simulink model "SWC_FDC_type"  (R2021b)
settings: Solver=FixedStepDiscrete  StartTime=0.0  StopTime=10.0  FixedStep=0.001  RelTol=1e-3
values from neighbouring files (symbols this model uses):
  DID_VCUKey = uint16(0x0202)    [vcu_local_hdr.m]
  DID_XWD = uint16(513)    [vcu_local_hdr.m]
  DIDLen_APSFunConfig = uint16(16)    [vcu_local_hdr.m]
  DIDLen_AutoLock = uint16(1)    [vcu_local_hdr.m]
  DIDLen_DKCKey = uint16(8)    [vcu_local_hdr.m]
  DIDLen_DRLDis = uint16(1)    [vcu_local_hdr.m]
  DIDLen_DynoMode = uint16(1)    [vcu_local_hdr.m]
  DIDLen_FMHTimer = uint16(1)    [vcu_local_hdr.m]
  DIDLen_LFLowPresThre = uint16(1)    [vcu_local_hdr.m]
  DIDLen_LFSensorID = uint16(4)    [vcu_local_hdr.m]
  DIDLen_LRLowPresThre = uint16(1)    [vcu_local_hdr.m]
  DIDLen_LRSensorID = uint16(4)    [vcu_local_hdr.m]
  DIDLen_RFLowPresThre = uint16(1)    [vcu_local_hdr.m]
  DIDLen_RFSensorID = uint16(4)    [vcu_local_hdr.m]
  DIDLen_RRLowPresThre = uint16(1)    [vcu_local_hdr.m]
  DIDLen_RRSensorID = uint16(4)    [vcu_local_hdr.m]
  DIDLen_SensorMode = uint16(1)    [vcu_local_hdr.m]
  DIDLen_TireSize = uint16(16)    [vcu_local_hdr.m]
  DIDLen_TPMSLearnSta = uint16(1)    [vcu_local_hdr.m]
  DIDLen_TurnLampFLThreCurr = uint16(1)    [vcu_local_hdr.m]
  DIDLen_TurnLampFRThreCurr = uint16(1)    [vcu_local_hdr.m]
  DIDLen_TurnLampRLThreCurr = uint16(1)    [vcu_local_hdr.m]
  DIDLen_TurnLampRRThreCurr = uint16(1)    [vcu_local_hdr.m]
  DIDLen_USSConfig = uint16(16)    [vcu_local_hdr.m]
  DIDLen_WhlPres = uint16(4)    [vcu_local_hdr.m]
  DIDLen_WhlSensorBattSta = uint16(1)    [vcu_local_hdr.m]
  DIDLen_WhlTmp = uint16(4)    [vcu_local_hdr.m]
  DIDLen_XWDMode = uint16(1)    [vcu_local_hdr.m]
  DIDNum_APSFunConfig = uint16(0x0903)    [vcu_local_hdr.m]
  DIDNum_AutoLock = uint16(0x0306)    [vcu_local_hdr.m]
  DIDNum_DKCKey = uint16(0x0202)    [vcu_local_hdr.m]
  DIDNum_DRLDis = uint16(0x0307)    [vcu_local_hdr.m]
  DIDNum_DynoMode = uint16(0x0203)    [vcu_local_hdr.m]
  DIDNum_FMHTimer = uint16(0x0305)    [vcu_local_hdr.m]
  DIDNum_LFLowPresThre = uint16(0x0B08)    [vcu_local_hdr.m]
  DIDNum_LFSensorID = uint16(0x0B01)    [vcu_local_hdr.m]
  DIDNum_LRLowPresThre = uint16(0x0B0A)    [vcu_local_hdr.m]
  DIDNum_LRSensorID = uint16(0x0B03)    [vcu_local_hdr.m]
  DIDNum_RFLowPresThre = uint16(0x0B09)    [vcu_local_hdr.m]
  DIDNum_RFSensorID = uint16(0x0B02)    [vcu_local_hdr.m]
  DIDNum_RRLowPresThre = uint16(0x0B0B)    [vcu_local_hdr.m]
  DIDNum_RRSensorID = uint16(0x0B04)    [vcu_local_hdr.m]
  DIDNum_SensorMode = uint16(0x0B0C)    [vcu_local_hdr.m]
  DIDNum_TireSize = uint16(0x0902)    [vcu_local_hdr.m]
  DIDNum_TPMSLearnSta = uint16(0x0B0D)    [vcu_local_hdr.m]
  DIDNum_TurnLampFLThreCurr = uint16(0x0303)    [vcu_local_hdr.m]
  DIDNum_TurnLampFRThreCurr = uint16(0x0301)    [vcu_local_hdr.m]
  DIDNum_TurnLampRLThreCurr = uint16(0x0304)    [vcu_local_hdr.m]
  DIDNum_TurnLampRRThreCurr = uint16(0x0302)    [vcu_local_hdr.m]
  DIDNum_USSConfig = uint16(0x0901)    [vcu_local_hdr.m]
  DIDNum_WhlPres = uint16(0x0B05)    [vcu_local_hdr.m]
  DIDNum_WhlSensorBattSta = uint16(0x0B07)    [vcu_local_hdr.m]
  DIDNum_WhlTmp = uint16(0x0B06)    [vcu_local_hdr.m]
  DIDNum_XWDMode = uint16(0x0201)    [vcu_local_hdr.m]
  DIDVCUKeyLength = uint16(8)    [vcu_local_hdr.m]
  ENUM_DRIVETRAIN_AWD = uint8(  2  )    [vcu_local_hdr.m]
  ENUM_DRIVETRAIN_FWD = uint8(  1  )    [vcu_local_hdr.m]
  ENUM_DRIVETRAIN_RWD = uint8(  0  )    [vcu_local_hdr.m]
  ENUM_TPMSLearnStatus_LEARNED = uint8(  1  )    [vcu_local_hdr.m]
  ENUM_TPMSLearnStatus_LEARNFAIL = uint8(  2  )    [vcu_local_hdr.m]
  ENUM_TPMSLearnStatus_NOTLEARN = uint8(  0  )    [vcu_local_hdr.m]
  ENUM_TPMSSTA_FAT = uint8(  8  )    [vcu_local_hdr.m]
  ENUM_TPMSSTA_LOWBATTERY = uint8(  2  )    [vcu_local_hdr.m]
  FALSE = boolean( 0 )    [vcu_local_hdr.m]
  ONE_INT = uint8(1)    [vcu_local_hdr.m]
  P_boolean = 0.0    [APPTypes.sldd]
  TRUE = boolean( 1 )    [vcu_local_hdr.m]
  ZERO_FLOAT = single(0)    [vcu_local_hdr.m]
  ZERO_INT = uint8(0)    [vcu_local_hdr.m]
undefined symbols (not defined in the file or in its folder): f32_ApsOutVehSpdSig, KHAL_DKCDecryptEnable_flg_ovrdflg, KHAL_DKCDecryptEnable_flg_ovrdval, KHAL_RandomNumberY1_enum, KHAL_RandomNumberY2_enum, KHAL_RandomNumberY_ovrdflg, KHAL_TPMSRESBUTT_flg_ovrdflg, KHAL_TPMSRESBUTT_flg_ovrdval, R_DIDWriteCDD_CSOP_DIDSet_APSFunConfig, R_DIDWriteCDD_CSOP_DIDSet_AutoLock, R_DIDWriteCDD_CSOP_DIDSet_DKCKey, R_DIDWriteCDD_CSOP_DIDSet_DRLDis, R_DIDWriteCDD_CSOP_DIDSet_DynoMode, R_DIDWriteCDD_CSOP_DIDSet_FMHTimer, R_DIDWriteCDD_CSOP_DIDSet_LFLowPresThre, R_DIDWriteCDD_CSOP_DIDSet_LFSensorID, R_DIDWriteCDD_CSOP_DIDSet_LRLowPresThre, R_DIDWriteCDD_CSOP_DIDSet_LRSensorID, R_DIDWriteCDD_CSOP_DIDSet_RFLowPresThre, R_DIDWriteCDD_CSOP_DIDSet_RFSensorID, R_DIDWriteCDD_CSOP_DIDSet_RRLowPresThre, R_DIDWriteCDD_CSOP_DIDSet_RRSensorID, R_DIDWriteCDD_CSOP_DIDSet_SensorMode, R_DIDWriteCDD_CSOP_DIDSet_TireSize, R_DIDWriteCDD_CSOP_DIDSet_TPMSLearnSta, R_DIDWriteCDD_CSOP_DIDSet_TurnLampFLThreCurr, R_DIDWriteCDD_CSOP_DIDSet_TurnLampFRThreCurr, R_DIDWriteCDD_CSOP_DIDSet_TurnLampRLThreCurr, R_DIDWriteCDD_CSOP_DIDSet_TurnLampRRThreCurr, R_DIDWriteCDD_CSOP_DIDSet_USSConfig, R_DIDWriteCDD_CSOP_DIDSet_WhlPres, R_DIDWriteCDD_CSOP_DIDSet_WhlSensorBattSta, R_DIDWriteCDD_CSOP_DIDSet_WhlTmp, R_DIDWriteCDD_CSOP_DIDSet_XWDMode, R_E2E_CAN3_VCU1_CSOP_Write_CAN3_VCU1, R_E2E_CAN3_VCU1_toNIDEC_CSOP_Write_CAN3_VCU1_toNIDEC, R_E2E_CAN4_VCU1_CSOP_Write_CAN4_VCU1, R_FDCCDD_Inner_CSOP_FDC_AppCallSleep, R_HALINCDD_CSOP_PAS_Handler, R_HALINCDD_CSOP_UDS_Main, R_HALOUT_APS_CSOP_ApsOutput, R_HALOUTCDD_CSOP_AppNmStateReq, R_HALOUTCDD_CSOP_SetAcoreRebootCmdACK, R_HALOUTCDD_CSOP_SetSysPwrStat, R_HALOUTCDD_CSOP_SleepRequest, R_IOExpOUT_CDD_CSOP_IOExpSetVal, R_J1939_CAN1_CFGEM1_BAM_CSOP_Write_CAN1_CFGEM1_BAM, R_J1939_CAN1_CFGEM1_DT_CSOP_Write_CAN1_CFGEM1_DT, R_NVMReadCDD_Inner_NVM_ReadOperation, R_NVMWriteCDD_Inner_NVM_WriteOperation, R_UDSCDD_CSOP_DdmRestartOperationCycle, R_WDGCDD_CSOP_Call_Watchdog, R_WDGCDD_CSOP_Call_WDG_AppEnd, R_WDGCDD_CSOP_Call_WDG_AppStart, u16_DIDLen_APSFunConfig, u16_DIDLen_AutoLock, u16_DIDLen_DKCKey, u16_DIDLen_DRLDis, u16_DIDLen_DynoMode, u16_DIDLen_FMHTimer ... (+83)
libraries: simulink x215, FVT_lib x143, hcu_lib x19, hdlsllib x9, app x1, halin x1, halout x1, inp x1, outp x1
(part 1 of 13)
settings Model: DataDictionary=APPTypes.sldd  Creator=FVT22063  LastModifiedBy=FVT22063
settings DataIOCC: SaveFormat=StructureWithTime
settings OptimizationCC: DefaultParameterBehavior=Inlined  EnhancedBackFolding=on  PassReuseOutputArgsAs=Individual arguments  ZeroExternalMemoryAtStartup=off  ZeroInternalMemoryAtStartup=off  OptimizeBlockOrder=speed  DifferentSizesBufferReuse=on  OptimizationCustomize=off  EfficientTunableParamExpr=on
settings DebuggingCC: ParameterTunabilityLossMsg=error
settings HardwareCC: ProdBitPerPointer=32  ProdBitPerSizeT=32  ProdBitPerPtrDiffT=32  ProdLargestAtomicInteger=Long  ProdLargestAtomicFloat=Double  ProdWordSize=32  ProdLongLongMode=on  ProdHWDeviceType=ARM Compatible->ARM Cortex-M
settings ModelReferenceCC: ModelReferenceNumInstancesAllowed=Single
settings SFSimCC: MATLABDynamicMemAlloc=off
settings RTWCC: Description=AUTOSAR  SystemTargetFile=autosar.tlc  GenCodeOnly=on  TemplateMakefile=ert_default_tmf  PortableWordSizes=on
settings CodeAppCC: ForceParamTrailComments=on  IgnoreCustomStorageClasses=off  OperatorAnnotations=on  SimulinkDataObjDesc=on  SFDataObjDesc=on  InsertBlockDesc=on
settings STFCustomTargetCC: TargetLangStandard=C99 (ISO)  MultiwordLength=256  ParMdlRefBuildCompliant=on  CompOptLevelCompliant=on  IncludeMdlTerminateFcn=off  CombineOutputUpdateFcns=on  SuppressErrorStatus=on  ERTCustomFileBanners=on  SupportNonFinite=off  SupportComplex=off  SupportContinuousTime=off  SupportNonInlinedSFcns=off  RemoveResetFunc=on  MATLABClassNameForMDSCustomization=Simulink.SoftwareTarget.ERTCustomization  AutosarCompliant=on  GRTInterface=off  UseToolchainInfoCompliant=on  LookupTableObjectStructAxisOrder=2,1,3,4,...  LUTObjectStructOrderEvenSpacing=Size,Table,Breakpoints  SystemTargetFile=autosar.tlc
settings ERTTargetCC: TargetLangStandard=C99 (ISO)  ConcurrentExecutionCompliant=off  IncludeMdlTerminateFcn=off  SuppressErrorStatus=on  SupportNonFinite=off  SupportComplex=off  ModelStepFunctionPrototypeControlCompliant=off  CPPClassGenCompliant=off  AutosarCompliant=on  LookupTableObjectStructAxisOrder=2,1,3,4,...  LUTObjectStructOrderEvenSpacing=Size,Table,Breakpoints  GenerateASAP2=on  InlinedParameterPlacement=NonHierarchical  ERTCustomFileTemplate=example_file_process.tlc  ConvertIfToSwitch=off  SuppressUnreachableDefaultCases=off  BooleanTrueId=true_MatlabRTW  BooleanFalseId=false_MatlabRTW

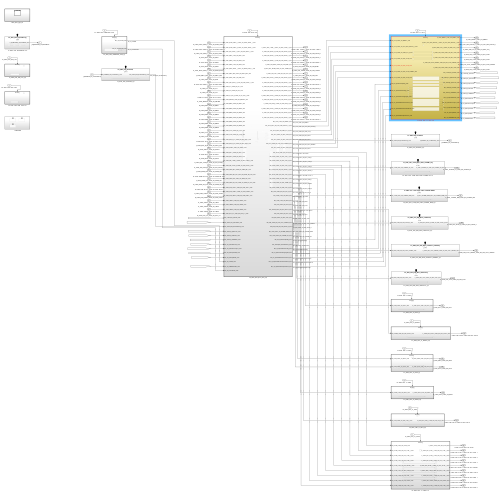
[thumbnail: Simulink's stored preview of the top-level diagram]
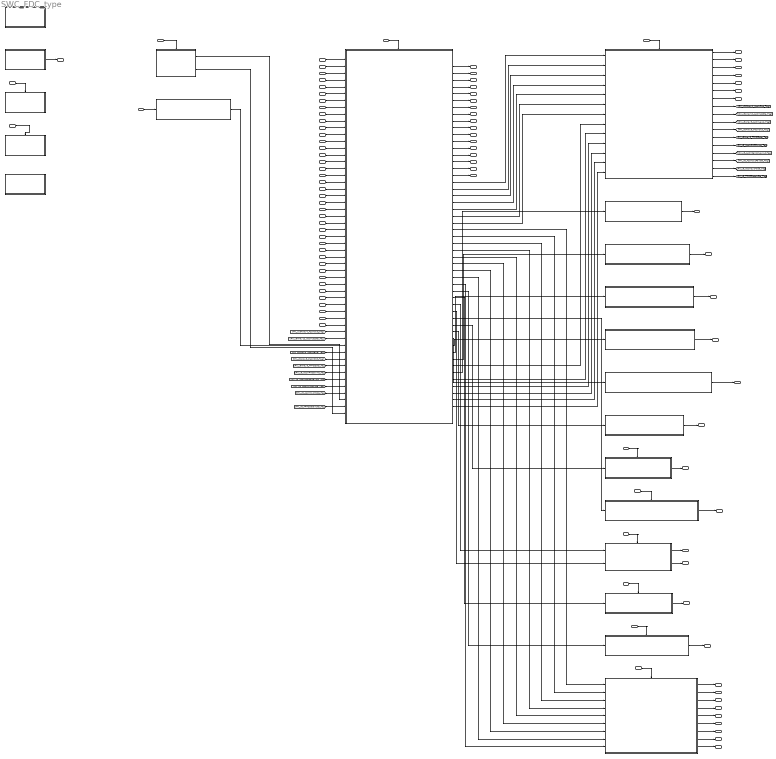
== system SWC_FDC_type ==
  run_SWC_FDC_PAS_1ms : Inport  SampleTime=0.001  OutputFunctionCall=on
  run_SWC_FDC_UDS_10ms : Inport  Port=2  SampleTime=0.01  OutputFunctionCall=on
  run_SWC_FDC_IOEXPCDD_10ms : Inport  Port=3  SampleTime=0.01  OutputFunctionCall=on
  run_SWC_FDC_RxTx_5ms : Inport  Port=4  SampleTime=0.005  OutputFunctionCall=on
  run_SWC_FDC_Tx_10ms : Inport  Port=5  SampleTime=0.01  OutputFunctionCall=on
  run_SWC_FDC_Tx_80ms : Inport  Port=6  SampleTime=0.08  OutputFunctionCall=on
  run_SWC_FDC_Tx_5000ms : Inport  Port=7  SampleTime=5  OutputFunctionCall=on
  run_SWC_FDC_Tx_50ms : Inport  Port=8  SampleTime=0.05  OutputFunctionCall=on
  run_SWC_FDC_Tx_250ms : Inport  Port=9  SampleTime=0.25  OutputFunctionCall=on
  run_SWC_FDC_Tx_20ms : Inport  Port=10  SampleTime=0.02  OutputFunctionCall=on
  run_SWC_FDC_Tx_100ms : Inport  Port=11  SampleTime=0.1  OutputFunctionCall=on
  R_NVMRead_NV_FVTDataArray : Inport  Port=12  OutDataTypeStr=uint8  PortDimensions=256
  R_CAN1_DCDC_Status_1_CAN1_SG_DCDC_Status_1 : Inport  Port=13  OutDataTypeStr=Bus: DT_CAN1_SG_DCDC_Status_1  PortDimensions=1  BusOutputAsStruct=on
  R_CAN1_DCDC_Status_2_CAN1_SG_DCDC_Status_2 : Inport  Port=14  OutDataTypeStr=Bus: DT_CAN1_SG_DCDC_Status_2  PortDimensions=1  BusOutputAsStruct=on
  R_CAN1_EAC_Status_1_CAN1_SG_EAC_Status_1 : Inport  Port=15  OutDataTypeStr=Bus: DT_CAN1_SG_EAC_Status_1  PortDimensions=1  BusOutputAsStruct=on
  R_CAN1_EBC1_CAN1_SG_EBC1 : Inport  Port=16  OutDataTypeStr=Bus: DT_CAN1_SG_EBC1  PortDimensions=1  BusOutputAsStruct=on
  R_CAN1_EBC2_CAN1_SG_EBC2 : Inport  Port=17  OutDataTypeStr=Bus: DT_CAN1_SG_EBC2  PortDimensions=1  BusOutputAsStruct=on
  R_CAN1_EBC5_CAN1_SG_EBC5 : Inport  Port=18  OutDataTypeStr=Bus: DT_CAN1_SG_EBC5  PortDimensions=1  BusOutputAsStruct=on
  R_CAN1_EHPS_Status_1_CAN1_SG_EHPS_Status_1 : Inport  Port=19  OutDataTypeStr=Bus: DT_CAN1_SG_EHPS_Status_1  PortDimensions=1  BusOutputAsStruct=on
  R_CAN1_EMC1_EM1_CAN1_SG_EMC1_EM1 : Inport  Port=20  OutDataTypeStr=Bus: DT_CAN1_SG_EMC1_EM1  PortDimensions=1  BusOutputAsStruct=on
  R_CAN1_EPB1_CAN1_SG_EPB1 : Inport  Port=21  OutDataTypeStr=Bus: DT_CAN1_SG_EPB1  PortDimensions=1  BusOutputAsStruct=on
  R_CAN1_PDU_Status_1_CAN1_SG_PDU_Status_1 : Inport  Port=22  OutDataTypeStr=Bus: DT_CAN1_SG_PDU_Status_1  PortDimensions=1  BusOutputAsStruct=on
  R_CAN2_IVI1_CAN2_SG_IVI1 : Inport  Port=23  OutDataTypeStr=Bus: DT_CAN2_SG_IVI1  PortDimensions=1  BusOutputAsStruct=on
  R_CAN2_IVI2_CAN2_SG_IVI2 : Inport  Port=24  OutDataTypeStr=Bus: DT_CAN2_SG_IVI2  PortDimensions=1  BusOutputAsStruct=on
  R_CAN2_IVI_P20_0_CAN2_SG_IVI_P20_0 : Inport  Port=25  OutDataTypeStr=Bus: DT_CAN2_SG_IVI_P20_0  PortDimensions=1  BusOutputAsStruct=on
  R_CAN2_METER1_CAN2_SG_METER1 : Inport  Port=26  OutDataTypeStr=Bus: DT_CAN2_SG_METER1  PortDimensions=1  BusOutputAsStruct=on
  R_CAN3_BMS1_CAN3_SG_BMS1 : Inport  Port=27  OutDataTypeStr=Bus: DT_CAN3_SG_BMS1  PortDimensions=1  BusOutputAsStruct=on
  R_CAN3_BMS3_CAN3_SG_BMS3 : Inport  Port=28  OutDataTypeStr=Bus: DT_CAN3_SG_BMS3  PortDimensions=1  BusOutputAsStruct=on
  R_CAN3_BMS4_CAN3_SG_BMS4 : Inport  Port=29  OutDataTypeStr=Bus: DT_CAN3_SG_BMS4  PortDimensions=1  BusOutputAsStruct=on
  R_CAN3_BMS5_CAN3_SG_BMS5 : Inport  Port=30  OutDataTypeStr=Bus: DT_CAN3_SG_BMS5  PortDimensions=1  BusOutputAsStruct=on
  R_CAN3_BMS6_CAN3_SG_BMS6 : Inport  Port=31  OutDataTypeStr=Bus: DT_CAN3_SG_BMS6  PortDimensions=1  BusOutputAsStruct=on
  R_CAN3_BMS8_CAN3_SG_BMS8 : Inport  Port=32  OutDataTypeStr=Bus: DT_CAN3_SG_BMS8  PortDimensions=1  BusOutputAsStruct=on
  R_CAN3_CCU1_CAN3_SG_CCU1 : Inport  Port=33  OutDataTypeStr=Bus: DT_CAN3_SG_CCU1  PortDimensions=1  BusOutputAsStruct=on
  R_CAN3_CCU2_CAN3_SG_CCU2 : Inport  Port=34  OutDataTypeStr=Bus: DT_CAN3_SG_CCU2  PortDimensions=1  BusOutputAsStruct=on
  R_CAN3_MCU_B_R1_CAN3_SG_MCU_B_R1 : Inport  Port=35  OutDataTypeStr=Bus: DT_CAN3_SG_MCU_B_R1  PortDimensions=1  BusOutputAsStruct=on
  R_CAN3_MCU_B_R2_CAN3_SG_MCU_B_R2 : Inport  Port=36  OutDataTypeStr=Bus: DT_CAN3_SG_MCU_B_R2  PortDimensions=1  BusOutputAsStruct=on
  R_CAN3_Shifter1_CAN3_SG_Shifter1 : Inport  Port=37  OutDataTypeStr=Bus: DT_CAN3_SG_Shifter1  PortDimensions=1  BusOutputAsStruct=on
  R_CAN4_DKC1_CAN4_SG_DKC1 : Inport  Port=38  OutDataTypeStr=Bus: DT_CAN4_SG_DKC1  PortDimensions=1  BusOutputAsStruct=on
  R_CAN4_DKC2_CAN4_SG_DKC2 : Inport  Port=39  OutDataTypeStr=Bus: DT_CAN4_SG_DKC2  PortDimensions=1  BusOutputAsStruct=on
  R_CAN4_Z24_C1000_0_CAN4_SG_Z24_C1000_0 : Inport  Port=40  OutDataTypeStr=Bus: DT_CAN4_SG_Z24_C1000_0  PortDimensions=1  BusOutputAsStruct=on
  R_CAN4_Z24_CE100_0_CAN4_SG_Z24_CE100_0 : Inport  Port=41  OutDataTypeStr=Bus: DT_CAN4_SG_Z24_CE100_0  PortDimensions=1  BusOutputAsStruct=on
  R_CAN4_ZONE_DR1_CAN4_SG_ZONE_DR1 : Inport  Port=42  OutDataTypeStr=Bus: DT_CAN4_SG_ZONE_DR1  PortDimensions=1  BusOutputAsStruct=on
  R_CAN4_ZONE_DR_VCU_CAN4_SG_ZONE_DR_VCU : Inport  Port=43  OutDataTypeStr=Bus: DT_CAN4_SG_ZONE_DR_VCU  PortDimensions=1  BusOutputAsStruct=on
  R_CAN4_ZONE_FR1_CAN4_SG_ZONE_FR1 : Inport  Port=44  OutDataTypeStr=Bus: DT_CAN4_SG_ZONE_FR1  PortDimensions=1  BusOutputAsStruct=on
  R_CAN4_ZONE_FR_VCU_CAN4_SG_ZONE_FR_VCU : Inport  Port=45  OutDataTypeStr=Bus: DT_CAN4_SG_ZONE_FR_VCU  PortDimensions=1  BusOutputAsStruct=on
  R_CAN4_zGW_APTC1_CAN4_SG_zGW_APTC1 : Inport  Port=46  OutDataTypeStr=Bus: DT_CAN4_SG_zGW_APTC1  PortDimensions=1  BusOutputAsStruct=on
  R_CAN4_zGW_CANFr1_CAN4_SG_zGW_CANFr1 : Inport  Port=47  OutDataTypeStr=Bus: DT_CAN4_SG_zGW_CANFr1  PortDimensions=1  BusOutputAsStruct=on
  R_CAN4_zGW_LINDr1_CAN4_SG_zGW_LINDr1 : Inport  Port=48  OutDataTypeStr=Bus: DT_CAN4_SG_zGW_LINDr1  PortDimensions=1  BusOutputAsStruct=on
  R_CAN5_TBOX1_CAN5_SG_TBOX1 : Inport  Port=49  OutDataTypeStr=Bus: DT_CAN5_SG_TBOX1  PortDimensions=1  BusOutputAsStruct=on
  R_CAN5_TBOX2_CAN5_SG_TBOX2 : Inport  Port=50  OutDataTypeStr=Bus: DT_CAN5_SG_TBOX2  PortDimensions=1  BusOutputAsStruct=on
  R_CAN5_TBOX3_CAN5_SG_TBOX3 : Inport  Port=51  OutDataTypeStr=Bus: DT_CAN5_SG_TBOX3  PortDimensions=1  BusOutputAsStruct=on
  R_CAN7_Door_Fr1_CAN7_SG_Door_Fr1 : Inport  Port=52  OutDataTypeStr=Bus: DT_CAN7_SG_Door_Fr1  PortDimensions=1  BusOutputAsStruct=on
  P_WDGCDD : Subsystem
  SWC_FDC_type_Init : Subsystem
  run_SWC_FDC_AppCallSleep_sys : Subsystem
  run_SWC_FDC_E2E_Write_CAN3VCU1_sys : Subsystem
  run_SWC_FDC_E2E_Write_CAN3VCU1_toNIDEC_sys : Subsystem
  run_SWC_FDC_E2E_Write_CAN4VCU1_sys : Subsystem
  run_SWC_FDC_IOEXPCDD_10ms_sys : Subsystem
  run_SWC_FDC_J1939_Write_CAN1_CFGEM1_BAM_sys : Subsystem
  run_SWC_FDC_J1939_Write_CAN1_CFGEM1_DT_sys : Subsystem
  run_SWC_FDC_NvmRead_sys : Subsystem
  run_SWC_FDC_NvmWrite_sys : Subsystem
  run_SWC_FDC_PAS_1ms_sys : Subsystem
  run_SWC_FDC_RxTx_5ms_sys : Subsystem
  run_SWC_FDC_Tx_100ms_sys : Subsystem
  run_SWC_FDC_Tx_10ms_sys : Subsystem
  run_SWC_FDC_Tx_20ms_sys : Subsystem
  run_SWC_FDC_Tx_250ms_sys : Subsystem
  run_SWC_FDC_Tx_5000ms_sys : Subsystem
  run_SWC_FDC_Tx_50ms_sys : Subsystem
  run_SWC_FDC_Tx_80ms_sys : Subsystem
  run_SWC_FDC_UDS_10ms_sys : Subsystem
  P_AppModeReq_requestedMode : Outport  OutDataTypeStr=Enum: AppModeRequestType  PortDimensions=1
  P_CAN1_GW1_C1000_1_CAN1_SG_GW1_C1000_1 : Outport  Port=2  OutDataTypeStr=Bus: DT_CAN1_SG_GW1_C1000_1  PortDimensions=1  BusOutputAsStruct=on
  P_CAN2_FD2_CE100_0_CAN2_SG_FD2_CE100_0 : Outport  Port=3  OutDataTypeStr=Bus: DT_CAN2_SG_FD2_CE100_0  PortDimensions=1  BusOutputAsStruct=on
  P_CAN2_FD2_CE100_1_CAN2_SG_FD2_CE100_1 : Outport  Port=4  OutDataTypeStr=Bus: DT_CAN2_SG_FD2_CE100_1  PortDimensions=1  BusOutputAsStruct=on
  P_CAN2_FD2_CE200_1_CAN2_SG_FD2_CE200_1 : Outport  Port=5  OutDataTypeStr=Bus: DT_CAN2_SG_FD2_CE200_1  PortDimensions=1  BusOutputAsStruct=on
  P_CAN3_FD3_BCM1_CAN3_SG_FD3_BCM1 : Outport  Port=6  OutDataTypeStr=Bus: DT_CAN3_SG_FD3_BCM1  PortDimensions=1  BusOutputAsStruct=on
  P_CAN3_FD3_THCM2_CAN3_SG_FD3_THCM2 : Outport  Port=7  OutDataTypeStr=Bus: DT_CAN3_SG_FD3_THCM2  PortDimensions=1  BusOutputAsStruct=on
  P_CAN3_FD3_V2L1_CAN3_SG_FD3_V2L1 : Outport  Port=8  OutDataTypeStr=Bus: DT_CAN3_SG_FD3_V2L1  PortDimensions=1  BusOutputAsStruct=on
  P_CAN3_GW3_CE100_0_CAN3_SG_GW3_CE100_0 : Outport  Port=9  OutDataTypeStr=Bus: DT_CAN3_SG_GW3_CE100_0  PortDimensions=1  BusOutputAsStruct=on
  P_CAN4_FD4_CE100_1_CAN4_SG_FD4_CE100_1 : Outport  Port=10  OutDataTypeStr=Bus: DT_CAN4_SG_FD4_CE100_1  PortDimensions=1  BusOutputAsStruct=on
  P_CAN4_FD4_CE100_3_CAN4_SG_FD4_CE100_3 : Outport  Port=11  OutDataTypeStr=Bus: DT_CAN4_SG_FD4_CE100_3  PortDimensions=1  BusOutputAsStruct=on
  P_CAN4_FD4_CE200_0_CAN4_SG_FD4_CE200_0 : Outport  Port=12  OutDataTypeStr=Bus: DT_CAN4_SG_FD4_CE200_0  PortDimensions=1  BusOutputAsStruct=on
  P_CAN4_GW4_CE100_0_CAN4_SG_GW4_CE100_0 : Outport  Port=13  OutDataTypeStr=Bus: DT_CAN4_SG_GW4_CE100_0  PortDimensions=1  BusOutputAsStruct=on
  P_CAN5_FD5_CE100_0_CAN5_SG_FD5_CE100_0 : Outport  Port=14  OutDataTypeStr=Bus: DT_CAN5_SG_FD5_CE100_0  PortDimensions=1  BusOutputAsStruct=on
  P_CAN5_FD5_Debug1_CAN5_SG_FD5_Debug1 : Outport  Port=15  OutDataTypeStr=Bus: DT_CAN5_SG_FD5_Debug1  PortDimensions=1  BusOutputAsStruct=on
  P_CAN5_GW5_CE100_0_CAN5_SG_GW5_CE100_0 : Outport  Port=16  OutDataTypeStr=Bus: DT_CAN5_SG_GW5_CE100_0  PortDimensions=1  BusOutputAsStruct=on
  P_CAN7_FD7_CE100_0_CAN7_SG_FD7_CE100_0 : Outport  Port=17  OutDataTypeStr=Bus: DT_CAN7_SG_FD7_CE100_0  PortDimensions=1  BusOutputAsStruct=on
  P_CAN7_FD7_CE100_1_CAN7_SG_FD7_CE100_1 : Outport  Port=18  OutDataTypeStr=Bus: DT_CAN7_SG_FD7_CE100_1  PortDimensions=1  BusOutputAsStruct=on
  P_CAN1_EMRC1_CAN1_SG_EMRC1 : Outport  Port=19  OutDataTypeStr=Bus: DT_CAN1_SG_EMRC1  PortDimensions=1  BusOutputAsStruct=on
  P_CAN1_VCU_PDU_Demand_1_CAN1_SG_VCU_PDU_Demand_1 : Outport  Port=20  OutDataTypeStr=Bus: DT_CAN1_SG_VCU_PDU_Demand_1  PortDimensions=1  BusOutputAsStruct=on
  P_CAN2_GW2_C10_0_CAN2_SG_GW2_C10_0 : Outport  Port=21  OutDataTypeStr=Bus: DT_CAN2_SG_GW2_C10_0  PortDimensions=1  BusOutputAsStruct=on
  P_CAN3_FD3_VCU0_CAN3_SG_FD3_VCU0 : Outport  Port=22  OutDataTypeStr=Bus: DT_CAN3_SG_FD3_VCU0  PortDimensions=1  BusOutputAsStruct=on
  P_CAN3_FD3_VCU2_CAN3_SG_FD3_VCU2 : Outport  Port=23  OutDataTypeStr=Bus: DT_CAN3_SG_FD3_VCU2  PortDimensions=1  BusOutputAsStruct=on
  P_CAN3_FD3_VCU2_toNIDEC_CAN3_SG_FD3_VCU2_toNIDEC : Outport  Port=24  OutDataTypeStr=Bus: DT_CAN3_SG_FD3_VCU2_toNIDEC  PortDimensions=1  BusOutputAsStruct=on
  P_CAN3_FD3_VCU5_CAN3_SG_FD3_VCU5 : Outport  Port=25  OutDataTypeStr=Bus: DT_CAN3_SG_FD3_VCU5  PortDimensions=1  BusOutputAsStruct=on
  P_NVMWrite_NV_FVTDataArray : Outport  Port=26  OutDataTypeStr=uint8  PortDimensions=256
  P_CAN1_CFGEM1_DT_CAN1_SG_CFGEM1_DT : Outport  Port=27  OutDataTypeStr=Bus: DT_CAN1_SG_CFGEM1_DT  PortDimensions=1  BusOutputAsStruct=on
  P_CAN1_CFGEM1_BAM_CAN1_SG_CFGEM1_BAM : Outport  Port=28  OutDataTypeStr=Bus: DT_CAN1_SG_CFGEM1_BAM  PortDimensions=1  BusOutputAsStruct=on
  P_CAN4_FD4_CE100_0_CAN4_SG_FD4_CE100_0 : Outport  Port=29  OutDataTypeStr=Bus: DT_CAN4_SG_FD4_CE100_0  PortDimensions=1  BusOutputAsStruct=on
  P_CAN3_FD3_VCU1_toNIDEC_CAN3_SG_FD3_VCU1_toNIDEC : Outport  Port=30  OutDataTypeStr=Bus: DT_CAN3_SG_FD3_VCU1_toNIDEC  PortDimensions=1  BusOutputAsStruct=on
  P_CAN3_FD3_VCU1_CAN3_SG_FD3_VCU1 : Outport  Port=31  OutDataTypeStr=Bus: DT_CAN3_SG_FD3_VCU1  PortDimensions=1  BusOutputAsStruct=on
  P_CAN1_ETC1_CAN1_SG_ETC1 : Outport  Port=32  OutDataTypeStr=Bus: DT_CAN1_SG_ETC1  PortDimensions=1  BusOutputAsStruct=on
  P_CAN2_FD2_Version_CAN2_SG_FD2_Version : Outport  Port=33  OutDataTypeStr=Bus: DT_CAN2_SG_FD2_Version  PortDimensions=1  BusOutputAsStruct=on
  P_CAN1_EEC2_CAN1_SG_EEC2 : Outport  Port=34  OutDataTypeStr=Bus: DT_CAN1_SG_EEC2  PortDimensions=1  BusOutputAsStruct=on
  P_CAN1_ETC2_CAN1_SG_ETC2 : Outport  Port=35  OutDataTypeStr=Bus: DT_CAN1_SG_ETC2  PortDimensions=1  BusOutputAsStruct=on
  P_CAN1_EEC3_CAN1_SG_EEC3 : Outport  Port=36  OutDataTypeStr=Bus: DT_CAN1_SG_EEC3  PortDimensions=1  BusOutputAsStruct=on
  P_CAN2_FD2_C20_0_CAN2_SG_FD2_C20_0 : Outport  Port=37  OutDataTypeStr=Bus: DT_CAN2_SG_FD2_C20_0  PortDimensions=1  BusOutputAsStruct=on
  P_CAN1_CCVS_CAN1_SG_CCVS : Outport  Port=38  OutDataTypeStr=Bus: DT_CAN1_SG_CCVS  PortDimensions=1  BusOutputAsStruct=on
  P_CAN1_FD1_C100_1_CAN1_SG_FD1_C100_1 : Outport  Port=39  OutDataTypeStr=Bus: DT_CAN1_SG_FD1_C100_1  PortDimensions=1  BusOutputAsStruct=on
  P_CAN1_FD1_C100_2_CAN1_SG_FD1_C100_2 : Outport  Port=40  OutDataTypeStr=Bus: DT_CAN1_SG_FD1_C100_2  PortDimensions=1  BusOutputAsStruct=on
  P_CAN1_FD1_C100_3_CAN1_SG_FD1_C100_3 : Outport  Port=41  OutDataTypeStr=Bus: DT_CAN1_SG_FD1_C100_3  PortDimensions=1  BusOutputAsStruct=on
  P_CAN1_FD1_CE100_1_CAN1_SG_FD1_CE100_1 : Outport  Port=42  OutDataTypeStr=Bus: DT_CAN1_SG_FD1_CE100_1  PortDimensions=1  BusOutputAsStruct=on
  P_CAN1_GW1_C100_4_CAN1_SG_GW1_C100_4 : Outport  Port=43  OutDataTypeStr=Bus: DT_CAN1_SG_GW1_C100_4  PortDimensions=1  BusOutputAsStruct=on
  P_CAN2_FD2_C200_1_CAN2_SG_FD2_C200_1 : Outport  Port=44  OutDataTypeStr=Bus: DT_CAN2_SG_FD2_C200_1  PortDimensions=1  BusOutputAsStruct=on
  P_CAN3_FD3_THCM1_CAN3_SG_FD3_THCM1 : Outport  Port=45  OutDataTypeStr=Bus: DT_CAN3_SG_FD3_THCM1  PortDimensions=1  BusOutputAsStruct=on
  P_CAN4_FD4_C100_0_CAN4_SG_FD4_C100_0 : Outport  Port=46  OutDataTypeStr=Bus: DT_CAN4_SG_FD4_C100_0  PortDimensions=1  BusOutputAsStruct=on
  wires:
  run_SWC_FDC_AppCallSleep_sys/1(P_AppModeReq_requestedMode_write) -> P_AppModeReq_requestedMode/1
  R_NVMRead_NV_FVTDataArray/1 -> run_SWC_FDC_NvmRead_sys/1(R_NVMRead_NV_FVTDataArray_read)
  R_CAN1_DCDC_Status_1_CAN1_SG_DCDC_Status_1/1 -> run_SWC_FDC_RxTx_5ms_sys/1(R_CAN1_DCDC_Status_1_CAN1_SG_DCDC_Status_1_read)
  R_CAN1_DCDC_Status_2_CAN1_SG_DCDC_Status_2/1 -> run_SWC_FDC_RxTx_5ms_sys/2(R_CAN1_DCDC_Status_2_CAN1_SG_DCDC_Status_2_read)
  R_CAN1_EAC_Status_1_CAN1_SG_EAC_Status_1/1 -> run_SWC_FDC_RxTx_5ms_sys/3(R_CAN1_EAC_Status_1_CAN1_SG_EAC_Status_1_read)
  R_CAN1_EBC1_CAN1_SG_EBC1/1 -> run_SWC_FDC_RxTx_5ms_sys/4(R_CAN1_EBC1_CAN1_SG_EBC1_read)
  R_CAN1_EBC2_CAN1_SG_EBC2/1 -> run_SWC_FDC_RxTx_5ms_sys/5(R_CAN1_EBC2_CAN1_SG_EBC2_read)
  R_CAN1_EBC5_CAN1_SG_EBC5/1 -> run_SWC_FDC_RxTx_5ms_sys/6(R_CAN1_EBC5_CAN1_SG_EBC5_read)
  R_CAN1_EHPS_Status_1_CAN1_SG_EHPS_Status_1/1 -> run_SWC_FDC_RxTx_5ms_sys/7(R_CAN1_EHPS_Status_1_CAN1_SG_EHPS_Status_1_read)
  R_CAN1_EMC1_EM1_CAN1_SG_EMC1_EM1/1 -> run_SWC_FDC_RxTx_5ms_sys/8(R_CAN1_EMC1_EM1_CAN1_SG_EMC1_EM1_read)
  R_CAN1_EPB1_CAN1_SG_EPB1/1 -> run_SWC_FDC_RxTx_5ms_sys/9(R_CAN1_EPB1_CAN1_SG_EPB1_read)
  R_CAN1_PDU_Status_1_CAN1_SG_PDU_Status_1/1 -> run_SWC_FDC_RxTx_5ms_sys/10(R_CAN1_PDU_Status_1_CAN1_SG_PDU_Status_1_read)
  R_CAN2_IVI1_CAN2_SG_IVI1/1 -> run_SWC_FDC_RxTx_5ms_sys/11(R_CAN2_IVI1_CAN2_SG_IVI1_read)
  R_CAN2_IVI2_CAN2_SG_IVI2/1 -> run_SWC_FDC_RxTx_5ms_sys/12(R_CAN2_IVI2_CAN2_SG_IVI2_read)
  R_CAN2_IVI_P20_0_CAN2_SG_IVI_P20_0/1 -> run_SWC_FDC_RxTx_5ms_sys/13(R_CAN2_IVI_P20_0_CAN2_SG_IVI_P20_0_read)
  R_CAN2_METER1_CAN2_SG_METER1/1 -> run_SWC_FDC_RxTx_5ms_sys/14(R_CAN2_METER1_CAN2_SG_METER1_read)
  R_CAN3_BMS1_CAN3_SG_BMS1/1 -> run_SWC_FDC_RxTx_5ms_sys/15(R_CAN3_BMS1_CAN3_SG_BMS1_read)
  R_CAN3_BMS3_CAN3_SG_BMS3/1 -> run_SWC_FDC_RxTx_5ms_sys/16(R_CAN3_BMS3_CAN3_SG_BMS3_read)
  R_CAN3_BMS4_CAN3_SG_BMS4/1 -> run_SWC_FDC_RxTx_5ms_sys/17(R_CAN3_BMS4_CAN3_SG_BMS4_read)
  R_CAN3_BMS5_CAN3_SG_BMS5/1 -> run_SWC_FDC_RxTx_5ms_sys/18(R_CAN3_BMS5_CAN3_SG_BMS5_read)
  R_CAN3_BMS6_CAN3_SG_BMS6/1 -> run_SWC_FDC_RxTx_5ms_sys/19(R_CAN3_BMS6_CAN3_SG_BMS6_read)
  R_CAN3_BMS8_CAN3_SG_BMS8/1 -> run_SWC_FDC_RxTx_5ms_sys/20(R_CAN3_BMS8_CAN3_SG_BMS8_read)
  R_CAN3_CCU1_CAN3_SG_CCU1/1 -> run_SWC_FDC_RxTx_5ms_sys/21(R_CAN3_CCU1_CAN3_SG_CCU1_read)
  R_CAN3_CCU2_CAN3_SG_CCU2/1 -> run_SWC_FDC_RxTx_5ms_sys/22(R_CAN3_CCU2_CAN3_SG_CCU2_read)
  R_CAN3_MCU_B_R1_CAN3_SG_MCU_B_R1/1 -> run_SWC_FDC_RxTx_5ms_sys/23(R_CAN3_MCU_B_R1_CAN3_SG_MCU_B_R1_read)
  R_CAN3_MCU_B_R2_CAN3_SG_MCU_B_R2/1 -> run_SWC_FDC_RxTx_5ms_sys/24(R_CAN3_MCU_B_R2_CAN3_SG_MCU_B_R2_read)
  R_CAN3_Shifter1_CAN3_SG_Shifter1/1 -> run_SWC_FDC_RxTx_5ms_sys/25(R_CAN3_Shifter1_CAN3_SG_Shifter1_read)
  R_CAN4_DKC1_CAN4_SG_DKC1/1 -> run_SWC_FDC_RxTx_5ms_sys/26(R_CAN4_DKC1_CAN4_SG_DKC1_read)
  R_CAN4_DKC2_CAN4_SG_DKC2/1 -> run_SWC_FDC_RxTx_5ms_sys/27(R_CAN4_DKC2_CAN4_SG_DKC2_read)
  R_CAN4_Z24_C1000_0_CAN4_SG_Z24_C1000_0/1 -> run_SWC_FDC_RxTx_5ms_sys/28(R_CAN4_Z24_C1000_0_CAN4_SG_Z24_C1000_0_read)
  R_CAN4_Z24_CE100_0_CAN4_SG_Z24_CE100_0/1 -> run_SWC_FDC_RxTx_5ms_sys/29(R_CAN4_Z24_CE100_0_CAN4_SG_Z24_CE100_0_read)
  R_CAN4_ZONE_DR1_CAN4_SG_ZONE_DR1/1 -> run_SWC_FDC_RxTx_5ms_sys/30(R_CAN4_ZONE_DR1_CAN4_SG_ZONE_DR1_read)
  R_CAN4_ZONE_DR_VCU_CAN4_SG_ZONE_DR_VCU/1 -> run_SWC_FDC_RxTx_5ms_sys/31(R_CAN4_ZONE_DR_VCU_CAN4_SG_ZONE_DR_VCU_read)
  R_CAN4_ZONE_FR1_CAN4_SG_ZONE_FR1/1 -> run_SWC_FDC_RxTx_5ms_sys/32(R_CAN4_ZONE_FR1_CAN4_SG_ZONE_FR1_read)
  R_CAN4_ZONE_FR_VCU_CAN4_SG_ZONE_FR_VCU/1 -> run_SWC_FDC_RxTx_5ms_sys/33(R_CAN4_ZONE_FR_VCU_CAN4_SG_ZONE_FR_VCU_read)
  R_CAN4_zGW_APTC1_CAN4_SG_zGW_APTC1/1 -> run_SWC_FDC_RxTx_5ms_sys/34(R_CAN4_zGW_APTC1_CAN4_SG_zGW_APTC1_read)
  R_CAN4_zGW_CANFr1_CAN4_SG_zGW_CANFr1/1 -> run_SWC_FDC_RxTx_5ms_sys/35(R_CAN4_zGW_CANFr1_CAN4_SG_zGW_CANFr1_read)
  R_CAN4_zGW_LINDr1_CAN4_SG_zGW_LINDr1/1 -> run_SWC_FDC_RxTx_5ms_sys/36(R_CAN4_zGW_LINDr1_CAN4_SG_zGW_LINDr1_read)
  R_CAN5_TBOX1_CAN5_SG_TBOX1/1 -> run_SWC_FDC_RxTx_5ms_sys/37(R_CAN5_TBOX1_CAN5_SG_TBOX1_read)
  R_CAN5_TBOX2_CAN5_SG_TBOX2/1 -> run_SWC_FDC_RxTx_5ms_sys/38(R_CAN5_TBOX2_CAN5_SG_TBOX2_read)
  R_CAN5_TBOX3_CAN5_SG_TBOX3/1 -> run_SWC_FDC_RxTx_5ms_sys/39(R_CAN5_TBOX3_CAN5_SG_TBOX3_read)
  R_CAN7_Door_Fr1_CAN7_SG_Door_Fr1/1 -> run_SWC_FDC_RxTx_5ms_sys/40(R_CAN7_Door_Fr1_CAN7_SG_Door_Fr1_read)
  run_SWC_FDC_RxTx_5ms_sys/1(P_CAN1_GW1_C1000_1_CAN1_SG_GW1_C1000_1_write) -> P_CAN1_GW1_C1000_1_CAN1_SG_GW1_C1000_1/1
  run_SWC_FDC_RxTx_5ms_sys/2(P_CAN2_FD2_CE100_0_CAN2_SG_FD2_CE100_0_write) -> P_CAN2_FD2_CE100_0_CAN2_SG_FD2_CE100_0/1
  run_SWC_FDC_RxTx_5ms_sys/3(P_CAN2_FD2_CE100_1_CAN2_SG_FD2_CE100_1_write) -> P_CAN2_FD2_CE100_1_CAN2_SG_FD2_CE100_1/1
  run_SWC_FDC_RxTx_5ms_sys/4(P_CAN2_FD2_CE200_1_CAN2_SG_FD2_CE200_1_write) -> P_CAN2_FD2_CE200_1_CAN2_SG_FD2_CE200_1/1
  run_SWC_FDC_RxTx_5ms_sys/5(P_CAN3_FD3_BCM1_CAN3_SG_FD3_BCM1_write) -> P_CAN3_FD3_BCM1_CAN3_SG_FD3_BCM1/1
  run_SWC_FDC_RxTx_5ms_sys/6(P_CAN3_FD3_THCM2_CAN3_SG_FD3_THCM2_write) -> P_CAN3_FD3_THCM2_CAN3_SG_FD3_THCM2/1
  run_SWC_FDC_RxTx_5ms_sys/7(P_CAN3_FD3_V2L1_CAN3_SG_FD3_V2L1_write) -> P_CAN3_FD3_V2L1_CAN3_SG_FD3_V2L1/1
  run_SWC_FDC_RxTx_5ms_sys/8(P_CAN3_GW3_CE100_0_CAN3_SG_GW3_CE100_0_write) -> P_CAN3_GW3_CE100_0_CAN3_SG_GW3_CE100_0/1
  run_SWC_FDC_RxTx_5ms_sys/9(P_CAN4_FD4_CE100_1_CAN4_SG_FD4_CE100_1_write) -> P_CAN4_FD4_CE100_1_CAN4_SG_FD4_CE100_1/1
  run_SWC_FDC_RxTx_5ms_sys/10(P_CAN4_FD4_CE100_3_CAN4_SG_FD4_CE100_3_write) -> P_CAN4_FD4_CE100_3_CAN4_SG_FD4_CE100_3/1
  run_SWC_FDC_RxTx_5ms_sys/11(P_CAN4_FD4_CE200_0_CAN4_SG_FD4_CE200_0_write) -> P_CAN4_FD4_CE200_0_CAN4_SG_FD4_CE200_0/1
  run_SWC_FDC_RxTx_5ms_sys/12(P_CAN4_GW4_CE100_0_CAN4_SG_GW4_CE100_0_write) -> P_CAN4_GW4_CE100_0_CAN4_SG_GW4_CE100_0/1
  run_SWC_FDC_RxTx_5ms_sys/13(P_CAN5_FD5_CE100_0_CAN5_SG_FD5_CE100_0_write) -> P_CAN5_FD5_CE100_0_CAN5_SG_FD5_CE100_0/1
  run_SWC_FDC_RxTx_5ms_sys/14(P_CAN5_FD5_Debug1_CAN5_SG_FD5_Debug1_write) -> P_CAN5_FD5_Debug1_CAN5_SG_FD5_Debug1/1
  run_SWC_FDC_RxTx_5ms_sys/15(P_CAN5_GW5_CE100_0_CAN5_SG_GW5_CE100_0_write) -> P_CAN5_GW5_CE100_0_CAN5_SG_GW5_CE100_0/1
  run_SWC_FDC_RxTx_5ms_sys/16(P_CAN7_FD7_CE100_0_CAN7_SG_FD7_CE100_0_write) -> P_CAN7_FD7_CE100_0_CAN7_SG_FD7_CE100_0/1
  run_SWC_FDC_RxTx_5ms_sys/17(P_CAN7_FD7_CE100_1_CAN7_SG_FD7_CE100_1_write) -> P_CAN7_FD7_CE100_1_CAN7_SG_FD7_CE100_1/1
  run_SWC_FDC_Tx_10ms_sys/1(P_CAN1_EMRC1_CAN1_SG_EMRC1_write) -> P_CAN1_EMRC1_CAN1_SG_EMRC1/1
  run_SWC_FDC_Tx_10ms_sys/2(P_CAN1_VCU_PDU_Demand_1_CAN1_SG_VCU_PDU_Demand_1_write) -> P_CAN1_VCU_PDU_Demand_1_CAN1_SG_VCU_PDU_Demand_1/1
  run_SWC_FDC_Tx_10ms_sys/3(P_CAN2_GW2_C10_0_CAN2_SG_GW2_C10_0_write) -> P_CAN2_GW2_C10_0_CAN2_SG_GW2_C10_0/1
  run_SWC_FDC_Tx_10ms_sys/4(P_CAN3_FD3_VCU0_CAN3_SG_FD3_VCU0_write) -> P_CAN3_FD3_VCU0_CAN3_SG_FD3_VCU0/1
  run_SWC_FDC_Tx_10ms_sys/5(P_CAN3_FD3_VCU2_CAN3_SG_FD3_VCU2_write) -> P_CAN3_FD3_VCU2_CAN3_SG_FD3_VCU2/1
  run_SWC_FDC_Tx_10ms_sys/6(P_CAN3_FD3_VCU2_toNIDEC_CAN3_SG_FD3_VCU2_toNIDEC_write) -> P_CAN3_FD3_VCU2_toNIDEC_CAN3_SG_FD3_VCU2_toNIDEC/1
  run_SWC_FDC_Tx_10ms_sys/7(P_CAN3_FD3_VCU5_CAN3_SG_FD3_VCU5_write) -> P_CAN3_FD3_VCU5_CAN3_SG_FD3_VCU5/1
  run_SWC_FDC_NvmWrite_sys/1(P_NVMWrite_NV_FVTDataArray_write) -> P_NVMWrite_NV_FVTDataArray/1
  run_SWC_FDC_J1939_Write_CAN1_CFGEM1_DT_sys/1(P_CAN1_CFGEM1_DT_CAN1_SG_CFGEM1_DT_write) -> P_CAN1_CFGEM1_DT_CAN1_SG_CFGEM1_DT/1
  run_SWC_FDC_J1939_Write_CAN1_CFGEM1_BAM_sys/1(P_CAN1_CFGEM1_BAM_CAN1_SG_CFGEM1_BAM_write) -> P_CAN1_CFGEM1_BAM_CAN1_SG_CFGEM1_BAM/1
  run_SWC_FDC_E2E_Write_CAN4VCU1_sys/1(P_CAN4_FD4_CE100_0_CAN4_SG_FD4_CE100_0_write) -> P_CAN4_FD4_CE100_0_CAN4_SG_FD4_CE100_0/1
  run_SWC_FDC_E2E_Write_CAN3VCU1_toNIDEC_sys/1(P_CAN3_FD3_VCU1_toNIDEC_CAN3_SG_FD3_VCU1_toNIDEC_write) -> P_CAN3_FD3_VCU1_toNIDEC_CAN3_SG_FD3_VCU1_toNIDEC/1
  run_SWC_FDC_E2E_Write_CAN3VCU1_sys/1(P_CAN3_FD3_VCU1_CAN3_SG_FD3_VCU1_write) -> P_CAN3_FD3_VCU1_CAN3_SG_FD3_VCU1/1
  run_SWC_FDC_Tx_80ms_sys/1(P_CAN1_ETC1_CAN1_SG_ETC1_write) -> P_CAN1_ETC1_CAN1_SG_ETC1/1
  run_SWC_FDC_Tx_5000ms_sys/1(P_CAN2_FD2_Version_CAN2_SG_FD2_Version_write) -> P_CAN2_FD2_Version_CAN2_SG_FD2_Version/1
  run_SWC_FDC_Tx_50ms_sys/1(P_CAN1_EEC2_CAN1_SG_EEC2_write) -> P_CAN1_EEC2_CAN1_SG_EEC2/1
  run_SWC_FDC_Tx_50ms_sys/2(P_CAN1_ETC2_CAN1_SG_ETC2_write) -> P_CAN1_ETC2_CAN1_SG_ETC2/1
  run_SWC_FDC_Tx_250ms_sys/1(P_CAN1_EEC3_CAN1_SG_EEC3_write) -> P_CAN1_EEC3_CAN1_SG_EEC3/1
  run_SWC_FDC_Tx_20ms_sys/1(P_CAN2_FD2_C20_0_CAN2_SG_FD2_C20_0_write) -> P_CAN2_FD2_C20_0_CAN2_SG_FD2_C20_0/1
  run_SWC_FDC_Tx_100ms_sys/1(P_CAN1_CCVS_CAN1_SG_CCVS_write) -> P_CAN1_CCVS_CAN1_SG_CCVS/1
  run_SWC_FDC_Tx_100ms_sys/2(P_CAN1_FD1_C100_1_CAN1_SG_FD1_C100_1_write) -> P_CAN1_FD1_C100_1_CAN1_SG_FD1_C100_1/1
  run_SWC_FDC_Tx_100ms_sys/3(P_CAN1_FD1_C100_2_CAN1_SG_FD1_C100_2_write) -> P_CAN1_FD1_C100_2_CAN1_SG_FD1_C100_2/1
  run_SWC_FDC_Tx_100ms_sys/4(P_CAN1_FD1_C100_3_CAN1_SG_FD1_C100_3_write) -> P_CAN1_FD1_C100_3_CAN1_SG_FD1_C100_3/1
  run_SWC_FDC_Tx_100ms_sys/5(P_CAN1_FD1_CE100_1_CAN1_SG_FD1_CE100_1_write) -> P_CAN1_FD1_CE100_1_CAN1_SG_FD1_CE100_1/1
  run_SWC_FDC_Tx_100ms_sys/6(P_CAN1_GW1_C100_4_CAN1_SG_GW1_C100_4_write) -> P_CAN1_GW1_C100_4_CAN1_SG_GW1_C100_4/1
  run_SWC_FDC_Tx_100ms_sys/7(P_CAN2_FD2_C200_1_CAN2_SG_FD2_C200_1_write) -> P_CAN2_FD2_C200_1_CAN2_SG_FD2_C200_1/1
  run_SWC_FDC_Tx_100ms_sys/8(P_CAN3_FD3_THCM1_CAN3_SG_FD3_THCM1_write) -> P_CAN3_FD3_THCM1_CAN3_SG_FD3_THCM1/1
  run_SWC_FDC_Tx_100ms_sys/9(P_CAN4_FD4_C100_0_CAN4_SG_FD4_C100_0_write) -> P_CAN4_FD4_C100_0_CAN4_SG_FD4_C100_0/1
  run_SWC_FDC_IOEXPCDD_10ms_sys/1(IRV_u8_CTDSW_write) -> run_SWC_FDC_RxTx_5ms_sys/51(IRV_u8_CTDSW_read)  "IRV_u8_CTDSW"
  run_SWC_FDC_IOEXPCDD_10ms_sys/2(IRV_u8_TrunkHanSW_write) -> run_SWC_FDC_RxTx_5ms_sys/53(IRV_u8_TrunkHanSW_read)  "IRV_u8_TrunkHanSW"
  run_SWC_FDC_NvmRead_sys/1(IRV_u8Array256_NvmReadArray_write) -> run_SWC_FDC_RxTx_5ms_sys/43(IRV_u8Array256_NvmReadArray_read)  "IRV_u8Array256_NvmReadArray"
  run_SWC_FDC_RxTx_5ms_sys/18(IRV_ms10_CAN1_SG_EMRC1_write) -> run_SWC_FDC_Tx_10ms_sys/1(IRV_ms10_CAN1_SG_EMRC1_read)  "IRV_ms10_CAN1_SG_EMRC1"
  run_SWC_FDC_RxTx_5ms_sys/19(IRV_ms10_CAN1_SG_VCU_PDU_Demand_1_write) -> run_SWC_FDC_Tx_10ms_sys/2(IRV_ms10_CAN1_SG_VCU_PDU_Demand_1_read)  "IRV_ms10_CAN1_SG_VCU_PDU_Demand_1"
  run_SWC_FDC_RxTx_5ms_sys/20(IRV_ms10_CAN2_SG_GW2_C10_0_write) -> run_SWC_FDC_Tx_10ms_sys/3(IRV_ms10_CAN2_SG_GW2_C10_0_read)  "IRV_ms10_CAN2_SG_GW2_C10_0"
  run_SWC_FDC_RxTx_5ms_sys/21(IRV_ms10_CAN3_SG_FD3_VCU0_write) -> run_SWC_FDC_Tx_10ms_sys/4(IRV_ms10_CAN3_SG_FD3_VCU0_read)  "IRV_ms10_CAN3_SG_FD3_VCU0"
  run_SWC_FDC_RxTx_5ms_sys/22(IRV_ms10_CAN3_SG_FD3_VCU2_write) -> run_SWC_FDC_Tx_10ms_sys/5(IRV_ms10_CAN3_SG_FD3_VCU2_read)  "IRV_ms10_CAN3_SG_FD3_VCU2"
  run_SWC_FDC_RxTx_5ms_sys/23(IRV_ms10_CAN3_SG_FD3_VCU2_toNIDEC_write) -> run_SWC_FDC_Tx_10ms_sys/6(IRV_ms10_CAN3_SG_FD3_VCU2_toNIDEC_read)  "IRV_ms10_CAN3_SG_FD3_VCU2_toNIDEC"
  run_SWC_FDC_RxTx_5ms_sys/24(IRV_ms10_CAN3_SG_FD3_VCU5_write) -> run_SWC_FDC_Tx_10ms_sys/7(IRV_ms10_CAN3_SG_FD3_VCU5_read)  "IRV_ms10_CAN3_SG_FD3_VCU5"
  run_SWC_FDC_RxTx_5ms_sys/25(IRV_ms100_CAN1_SG_CCVS_write) -> run_SWC_FDC_Tx_100ms_sys/1(IRV_ms100_CAN1_SG_CCVS_read)  "IRV_ms100_CAN1_SG_CCVS"
  run_SWC_FDC_RxTx_5ms_sys/26(IRV_ms100_CAN1_SG_FD1_C100_1_write) -> run_SWC_FDC_Tx_100ms_sys/2(IRV_ms100_CAN1_SG_FD1_C100_1_read)  "IRV_ms100_CAN1_SG_FD1_C100_1"
  run_SWC_FDC_RxTx_5ms_sys/27(IRV_ms100_CAN1_SG_FD1_C100_2_write) -> run_SWC_FDC_Tx_100ms_sys/3(IRV_ms100_CAN1_SG_FD1_C100_2_read)  "IRV_ms100_CAN1_SG_FD1_C100_2"
  run_SWC_FDC_RxTx_5ms_sys/28(IRV_ms100_CAN1_SG_FD1_C100_3_write) -> run_SWC_FDC_Tx_100ms_sys/4(IRV_ms100_CAN1_SG_FD1_C100_3_read)  "IRV_ms100_CAN1_SG_FD1_C100_3"
  run_SWC_FDC_RxTx_5ms_sys/29(IRV_ms100_CAN1_SG_FD1_CE100_1_write) -> run_SWC_FDC_Tx_100ms_sys/5(IRV_ms100_CAN1_SG_FD1_CE100_1_read)  "IRV_ms100_CAN1_SG_FD1_CE100_1"
  run_SWC_FDC_RxTx_5ms_sys/30(IRV_ms100_CAN1_SG_GW1_C100_4_write) -> run_SWC_FDC_Tx_100ms_sys/6(IRV_ms100_CAN1_SG_GW1_C100_4_read)  "IRV_ms100_CAN1_SG_GW1_C100_4"
  run_SWC_FDC_RxTx_5ms_sys/31(IRV_ms100_CAN2_SG_FD2_C200_1_write) -> run_SWC_FDC_Tx_100ms_sys/7(IRV_ms100_CAN2_SG_FD2_C200_1_read)  "IRV_ms100_CAN2_SG_FD2_C200_1"
  run_SWC_FDC_RxTx_5ms_sys/32(IRV_ms100_CAN3_SG_FD3_THCM1_write) -> run_SWC_FDC_Tx_100ms_sys/8(IRV_ms100_CAN3_SG_FD3_THCM1_read)  "IRV_ms100_CAN3_SG_FD3_THCM1"
  run_SWC_FDC_RxTx_5ms_sys/33(IRV_ms100_CAN4_SG_FD4_C100_0_write) -> run_SWC_FDC_Tx_100ms_sys/9(IRV_ms100_CAN4_SG_FD4_C100_0_read)  "IRV_ms100_CAN4_SG_FD4_C100_0"
  run_SWC_FDC_RxTx_5ms_sys/34(IRV_ms20_CAN2_SG_FD2_C20_0_write) -> run_SWC_FDC_Tx_20ms_sys/1(IRV_ms20_CAN2_SG_FD2_C20_0_read)  "IRV_ms20_CAN2_SG_FD2_C20_0"
  run_SWC_FDC_RxTx_5ms_sys/35(IRV_ms250_CAN1_SG_EEC3_write) -> run_SWC_FDC_Tx_250ms_sys/1(IRV_ms250_CAN1_SG_EEC3_read)  "IRV_ms250_CAN1_SG_EEC3"
  run_SWC_FDC_RxTx_5ms_sys/36(IRV_ms50_CAN1_SG_EEC2_write) -> run_SWC_FDC_Tx_50ms_sys/1(IRV_ms50_CAN1_SG_EEC2_read)  "IRV_ms50_CAN1_SG_EEC2"
  run_SWC_FDC_RxTx_5ms_sys/37(IRV_ms50_CAN1_SG_ETC2_write) -> run_SWC_FDC_Tx_50ms_sys/2(IRV_ms50_CAN1_SG_ETC2_read)  "IRV_ms50_CAN1_SG_ETC2"
  run_SWC_FDC_RxTx_5ms_sys/38(IRV_ms5000_CAN2_SG_FD2_Version_write) -> run_SWC_FDC_Tx_5000ms_sys/1(IRV_ms5000_CAN2_SG_FD2_Version_read)  "IRV_ms5000_CAN2_SG_FD2_Version"
  run_SWC_FDC_RxTx_5ms_sys/39(IRV_ms80_CAN1_SG_ETC1_write) -> run_SWC_FDC_Tx_80ms_sys/1(IRV_ms80_CAN1_SG_ETC1_read)  "IRV_ms80_CAN1_SG_ETC1"
  run_SWC_FDC_RxTx_5ms_sys/40(IRV_E2E_CAN3_SG_FD3_VCU1_write) -> run_SWC_FDC_E2E_Write_CAN3VCU1_sys/1(IRV_E2E_CAN3_SG_FD3_VCU1_read)  "IRV_E2E_CAN3_SG_FD3_VCU1"
  run_SWC_FDC_RxTx_5ms_sys/41(IRV_E2E_CAN3_SG_FD3_VCU1_toNIDEC_write) -> run_SWC_FDC_E2E_Write_CAN3VCU1_toNIDEC_sys/1(IRV_E2E_CAN3_SG_FD3_VCU1_toNIDEC_read)  "IRV_E2E_CAN3_SG_FD3_VCU1_toNIDEC"
  run_SWC_FDC_RxTx_5ms_sys/42(IRV_E2E_CAN4_SG_FD4_CE100_0_write) -> run_SWC_FDC_E2E_Write_CAN4VCU1_sys/1(IRV_E2E_CAN4_SG_FD4_CE100_0_read)  "IRV_E2E_CAN4_SG_FD4_CE100_0"
  run_SWC_FDC_RxTx_5ms_sys/43(IRV_J1939_CAN1_SG_CFGEM1_BAM_write) -> run_SWC_FDC_J1939_Write_CAN1_CFGEM1_BAM_sys/1(IRV_J1939_CAN1_SG_CFGEM1_BAM_read)  "IRV_J1939_CAN1_SG_CFGEM1_BAM"
  run_SWC_FDC_RxTx_5ms_sys/44(IRV_J1939_CAN1_SG_CFGEM1_DT_write) -> run_SWC_FDC_J1939_Write_CAN1_CFGEM1_DT_sys/1(IRV_J1939_CAN1_SG_CFGEM1_DT_read)  "IRV_J1939_CAN1_SG_CFGEM1_DT"
  run_SWC_FDC_RxTx_5ms_sys/45(IRV_f32_ApsOutVehSpdSig_write) -> run_SWC_FDC_Tx_10ms_sys/8(IRV_f32_ApsOutVehSpdSig_read)  "IRV_f32_ApsOutVehSpdSig"
  run_SWC_FDC_RxTx_5ms_sys/46(IRV_u8Array256_NvmWriteArray_write) -> run_SWC_FDC_NvmWrite_sys/1(IRV_u8Array256_NvmWriteArray_read)  "IRV_u8Array256_NvmWriteArray"
  run_SWC_FDC_RxTx_5ms_sys/47(IRV_u8_ApsOutGearPosnSig_write) -> run_SWC_FDC_Tx_10ms_sys/9(IRV_u8_ApsOutGearPosnSig_read)  "IRV_u8_ApsOutGearPosnSig"
  run_SWC_FDC_RxTx_5ms_sys/48(IRV_u8_ApsOutSendChrgPlugSta_write) -> run_SWC_FDC_Tx_10ms_sys/10(IRV_u8_ApsOutSendChrgPlugSta_read)  "IRV_u8_ApsOutSendChrgPlugSta"
  run_SWC_FDC_RxTx_5ms_sys/49(IRV_u8_ApsOutSetFrSensorOnCmd_write) -> run_SWC_FDC_Tx_10ms_sys/11(IRV_u8_ApsOutSetFrSensorOnCmd_read)  "IRV_u8_ApsOutSetFrSensorOnCmd"
  run_SWC_FDC_RxTx_5ms_sys/50(IRV_u8_ApsOutSetFrSensorSwTOCmd_write) -> run_SWC_FDC_Tx_10ms_sys/12(IRV_u8_ApsOutSetFrSensorSwTOCmd_read)  "IRV_u8_ApsOutSetFrSensorSwTOCmd"
  run_SWC_FDC_RxTx_5ms_sys/51(IRV_u8_ApsOutSetVehSpdTOCmd_write) -> run_SWC_FDC_Tx_10ms_sys/13(IRV_u8_ApsOutSetVehSpdTOCmd_read)  "IRV_u8_ApsOutSetVehSpdTOCmd"
  run_SWC_FDC_Tx_10ms_sys/17(IRV_u8_TPMSDataInSta_write) -> [IRV_u8_TPMSDataInSta_Tag]  "IRV_u8_TPMSDataInSta"
  [IRV_u8_TPMSDataInSta_Tag] -> run_SWC_FDC_RxTx_5ms_sys/52(IRV_u8_TPMSDataInSta_read)
  run_SWC_FDC_Tx_10ms_sys/16(IRV_u8_ApsInSysMode_write) -> [IRV_u8_ApsInSysMode_Tag]  "IRV_u8_ApsInSysMode"
  [IRV_u8_ApsInSysMode_Tag] -> run_SWC_FDC_RxTx_5ms_sys/50(IRV_u8_ApsInSysMode_read)
  run_SWC_FDC_Tx_10ms_sys/15(IRV_u8_ApsInSysFailSta_write) -> [IRV_u8_ApsInSysFailSta_Tag]  "IRV_u8_ApsInSysFailSta"
  [IRV_u8_ApsInSysFailSta_Tag] -> run_SWC_FDC_RxTx_5ms_sys/49(IRV_u8_ApsInSysFailSta_read)
  run_SWC_FDC_Tx_10ms_sys/14(IRV_u8_ApsInSensorLayout_write) -> [IRV_u8_ApsInSensorLayout_Tag]  "IRV_u8_ApsInSensorLayout"
  [IRV_u8_ApsInSensorLayout_Tag] -> run_SWC_FDC_RxTx_5ms_sys/48(IRV_u8_ApsInSensorLayout_read)
  run_SWC_FDC_Tx_10ms_sys/13(IRV_u8_ApsInPASChime_write) -> [IRV_u8_ApsInPASChime_Tag]  "IRV_u8_ApsInPASChime"
  [IRV_u8_ApsInPASChime_Tag] -> run_SWC_FDC_RxTx_5ms_sys/47(IRV_u8_ApsInPASChime_read)
  run_SWC_FDC_Tx_10ms_sys/12(IRV_u8Array9_TPMSData_write) -> [IRV_u8Array9_TPMSData_Tag]  "IRV_u8Array9_TPMSData"
  [IRV_u8Array9_TPMSData_Tag] -> run_SWC_FDC_RxTx_5ms_sys/46(IRV_u8Array9_TPMSData_read)
  run_SWC_FDC_Tx_10ms_sys/11(IRV_u8Array8_PasInDist_write) -> [IRV_u8Array8_PasInDist_Tag]  "IRV_u8Array8_PasInDist"
  [IRV_u8Array8_PasInDist_Tag] -> run_SWC_FDC_RxTx_5ms_sys/45(IRV_u8Array8_PasInDist_read)
  run_SWC_FDC_Tx_10ms_sys/10(IRV_u8Array8_ApsInLevel_write) -> [IRV_u8Array8_ApsInLevel_Tag]  "IRV_u8Array8_ApsInLevel"
  [IRV_u8Array8_ApsInLevel_Tag] -> run_SWC_FDC_RxTx_5ms_sys/44(IRV_u8Array8_ApsInLevel_read)
  run_SWC_FDC_Tx_10ms_sys/9(IRV_u8Array12_ApsInUssSta_write) -> [IRV_u8Array12_ApsInUssSta_Tag]  "IRV_u8Array12_ApsInUssSta"
  [IRV_u8Array12_ApsInUssSta_Tag] -> run_SWC_FDC_RxTx_5ms_sys/42(IRV_u8Array12_ApsInUssSta_read)
  run_SWC_FDC_Tx_10ms_sys/8(IRV_u16Array4_ApsInDist_write) -> [IRV_u16Array4_ApsInDist_Tag]  "IRV_u16Array4_ApsInDist"
  [IRV_u16Array4_ApsInDist_Tag] -> run_SWC_FDC_RxTx_5ms_sys/41(IRV_u16Array4_ApsInDist_read)
  run_SWC_FDC_PAS_1ms/1 -> run_SWC_FDC_PAS_1ms_sys/Trigger
  run_SWC_FDC_UDS_10ms/1 -> run_SWC_FDC_UDS_10ms_sys/Trigger
  run_SWC_FDC_IOEXPCDD_10ms/1 -> run_SWC_FDC_IOEXPCDD_10ms_sys/Trigger
  run_SWC_FDC_RxTx_5ms/1 -> run_SWC_FDC_RxTx_5ms_sys/Trigger
  run_SWC_FDC_Tx_10ms/1 -> run_SWC_FDC_Tx_10ms_sys/Trigger
  run_SWC_FDC_Tx_80ms/1 -> run_SWC_FDC_Tx_80ms_sys/Trigger
  run_SWC_FDC_Tx_5000ms/1 -> run_SWC_FDC_Tx_5000ms_sys/Trigger
  run_SWC_FDC_Tx_50ms/1 -> run_SWC_FDC_Tx_50ms_sys/Trigger
  run_SWC_FDC_Tx_250ms/1 -> run_SWC_FDC_Tx_250ms_sys/Trigger
  run_SWC_FDC_Tx_20ms/1 -> run_SWC_FDC_Tx_20ms_sys/Trigger
  run_SWC_FDC_Tx_100ms/1 -> run_SWC_FDC_Tx_100ms_sys/Trigger

== system SWC_FDC_type/P_WDGCDD ==
  run_SWC_FDC_AppCallWDG_End_sys : Subsystem
  run_SWC_FDC_AppCallWDG_StartUp_sys : Subsystem
  run_SWC_FDC_AppCallWDG_sys : Subsystem

== system SWC_FDC_type/SWC_FDC_type_Init ==
  Event Listener : EventListener  EventName=reset

== system SWC_FDC_type/run_SWC_FDC_AppCallSleep_sys ==
  function : TriggerPort  TriggerType=function-call  IsSimulinkFunction=on  FunctionName=run_SWC_FDC_AppCallSleep  VariantControl=(inherit)
  Constant : Constant  Value=TRUE
  Data Type Conversion : DataTypeConversion  OutDataTypeStr=Enum: AppModeRequestType
  Data Type Conversion1 : DataTypeConversion  OutDataTypeStr=uint8
  P_AppModeReq_requestedMode_write : Outport
  wires:
  Data Type Conversion/1 -> P_AppModeReq_requestedMode_write/1
  Data Type Conversion1/1 -> Data Type Conversion/1
  Constant/1 -> Data Type Conversion1/1

== system SWC_FDC_type/run_SWC_FDC_E2E_Write_CAN3VCU1_sys ==
  IRV_E2E_CAN3_SG_FD3_VCU1_read : Inport
  function : TriggerPort  TriggerType=function-call  IsSimulinkFunction=on  FunctionName=run_SWC_FDC_E2E_Write_CAN3VCU1  VariantControl=(inherit)
  P_CAN3_FD3_VCU1_CAN3_SG_FD3_VCU1_write : Outport
  wires:
  IRV_E2E_CAN3_SG_FD3_VCU1_read/1 -> P_CAN3_FD3_VCU1_CAN3_SG_FD3_VCU1_write/1

== system SWC_FDC_type/run_SWC_FDC_E2E_Write_CAN3VCU1_toNIDEC_sys ==
  IRV_E2E_CAN3_SG_FD3_VCU1_toNIDEC_read : Inport
  function : TriggerPort  TriggerType=function-call  IsSimulinkFunction=on  FunctionName=run_SWC_FDC_E2E_Write_CAN3VCU1_toNIDEC  VariantControl=(inherit)
  P_CAN3_FD3_VCU1_toNIDEC_CAN3_SG_FD3_VCU1_toNIDEC_write : Outport
  wires:
  IRV_E2E_CAN3_SG_FD3_VCU1_toNIDEC_read/1 -> P_CAN3_FD3_VCU1_toNIDEC_CAN3_SG_FD3_VCU1_toNIDEC_write/1

== system SWC_FDC_type/run_SWC_FDC_E2E_Write_CAN4VCU1_sys ==
  IRV_E2E_CAN4_SG_FD4_CE100_0_read : Inport
  function : TriggerPort  TriggerType=function-call  IsSimulinkFunction=on  FunctionName=run_SWC_FDC_E2E_Write_CAN4VCU1  VariantControl=(inherit)
  P_CAN4_FD4_CE100_0_CAN4_SG_FD4_CE100_0_write : Outport
  wires:
  IRV_E2E_CAN4_SG_FD4_CE100_0_read/1 -> P_CAN4_FD4_CE100_0_CAN4_SG_FD4_CE100_0_write/1

== system SWC_FDC_type/run_SWC_FDC_IOEXPCDD_10ms_sys ==
  function : TriggerPort  TriggerType=function-call  VariantControl=(inherit)  SampleTimeType=periodic  SampleTime=-1
  R_IOExpIN_CDD_CSOP_IOExpGetVal : FunctionCaller  FunctionPrototype=[u8_CTDSW,u8_TrunkHanSW] = R_IOExpIN_CDD_CSOP_IOExpGetVal()  OutputArgumentSpecifications=uint8(1), uint8(1)
  IRV_u8_CTDSW_write : Outport  OutDataTypeStr=uint8  PortDimensions=1
  IRV_u8_TrunkHanSW_write : Outport  Port=2  OutDataTypeStr=uint8  PortDimensions=1
  wires:
  R_IOExpIN_CDD_CSOP_IOExpGetVal/1 -> IRV_u8_CTDSW_write/1
  R_IOExpIN_CDD_CSOP_IOExpGetVal/2 -> IRV_u8_TrunkHanSW_write/1

== system SWC_FDC_type/run_SWC_FDC_J1939_Write_CAN1_CFGEM1_BAM_sys ==
  IRV_J1939_CAN1_SG_CFGEM1_BAM_read : Inport
  function : TriggerPort  TriggerType=function-call  IsSimulinkFunction=on  FunctionName=run_SWC_FDC_J1939_Write_CAN1_CFGEM1_BAM  VariantControl=(inherit)
  P_CAN1_CFGEM1_BAM_CAN1_SG_CFGEM1_BAM_write : Outport
  wires:
  IRV_J1939_CAN1_SG_CFGEM1_BAM_read/1 -> P_CAN1_CFGEM1_BAM_CAN1_SG_CFGEM1_BAM_write/1

== system SWC_FDC_type/run_SWC_FDC_J1939_Write_CAN1_CFGEM1_DT_sys ==
  IRV_J1939_CAN1_SG_CFGEM1_DT_read : Inport
  function : TriggerPort  TriggerType=function-call  IsSimulinkFunction=on  FunctionName=run_SWC_FDC_J1939_Write_CAN1_CFGEM1_DT  VariantControl=(inherit)
  P_CAN1_CFGEM1_DT_CAN1_SG_CFGEM1_DT_write : Outport
  wires:
  IRV_J1939_CAN1_SG_CFGEM1_DT_read/1 -> P_CAN1_CFGEM1_DT_CAN1_SG_CFGEM1_DT_write/1

== system SWC_FDC_type/run_SWC_FDC_NvmRead_sys ==
  R_NVMRead_NV_FVTDataArray_read : Inport
  function : TriggerPort  TriggerType=function-call  IsSimulinkFunction=on  FunctionName=run_SWC_FDC_NvmRead  VariantControl=(inherit)
  IRV_u8Array256_NvmReadArray_write : Outport  OutDataTypeStr=uint8  PortDimensions=256
  wires:
  R_NVMRead_NV_FVTDataArray_read/1 -> IRV_u8Array256_NvmReadArray_write/1

== system SWC_FDC_type/run_SWC_FDC_NvmWrite_sys ==
  IRV_u8Array256_NvmWriteArray_read : Inport
  function : TriggerPort  TriggerType=function-call  IsSimulinkFunction=on  FunctionName=run_SWC_FDC_NvmWrite  VariantControl=(inherit)
  P_NVMWrite_NV_FVTDataArray_write : Outport
  wires:
  IRV_u8Array256_NvmWriteArray_read/1 -> P_NVMWrite_NV_FVTDataArray_write/1

== system SWC_FDC_type/run_SWC_FDC_PAS_1ms_sys ==
  function : TriggerPort  TriggerType=function-call  VariantControl=(inherit)  SampleTimeType=periodic  SampleTime=-1
  R_HALINCDD_CSOP_PAS_Handler : FunctionCaller  FunctionPrototype=R_HALINCDD_CSOP_PAS_Handler()
